simulink model "P1_1_1"  (R2020a)
settings: Solver=VariableStepAuto  StartTime=0.0  StopTime=1  RelTol=1e-3
undefined symbols (not defined in the file): b, k, r
libraries: cstblocks x6
settings Model: Creator=beto1  LastModifiedBy=beto1

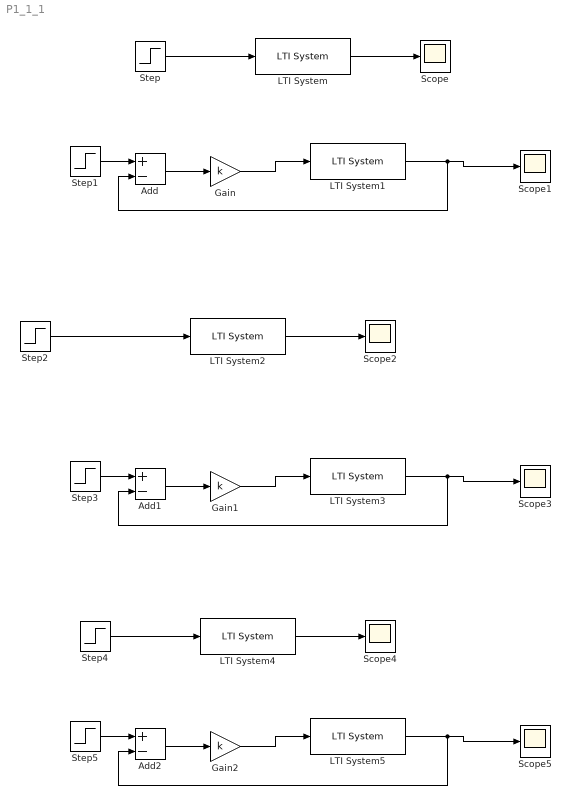
== system P1_1_1 ==
  Add : Sum  Inputs=+-
  Add1 : Sum  Inputs=+-
  Add2 : Sum  Inputs=+-
  Gain : Gain  Gain=k
  Gain1 : Gain  Gain=k
  Gain2 : Gain  Gain=k
  LTI System : cstblocks/LTI System  sys=G  IC=[]
  LTI System1 : cstblocks/LTI System  sys=G  IC=[]
  LTI System2 : cstblocks/LTI System  sys=G2  IC=[]
  LTI System3 : cstblocks/LTI System  sys=G2  IC=[]
  LTI System4 : cstblocks/LTI System  sys=G3  IC=[]
  LTI System5 : cstblocks/LTI System  sys=G3  IC=[]
  Scope{,1..5} (6 alike) : Scope
  Step : Step  Time=0  After=b  SampleTime=0
  Step1 : Step  Time=0  After=r  SampleTime=0
  Step2 : Step  Time=0  After=b  SampleTime=0
  Step3 : Step  Time=0  After=r  SampleTime=0
  Step4 : Step  Time=0  After=b  SampleTime=0
  Step5 : Step  Time=0  After=r  SampleTime=0
  wires:
  Step/1 -> LTI System/1
  LTI System/1 -> Scope/1
  LTI System1/1 -> Add/2, Scope1/1
  Add/1 -> Gain/1
  Gain/1 -> LTI System1/1
  Step1/1 -> Add/1
  Step2/1 -> LTI System2/1
  LTI System2/1 -> Scope2/1
  LTI System3/1 -> Add1/2, Scope3/1
  Step3/1 -> Add1/1
  Gain1/1 -> LTI System3/1
  Add1/1 -> Gain1/1
  LTI System4/1 -> Scope4/1
  Step4/1 -> LTI System4/1
  LTI System5/1 -> Add2/2, Scope5/1
  Add2/1 -> Gain2/1
  Step5/1 -> Add2/1
  Gain2/1 -> LTI System5/1
